simulink model "SoRo_Crt_SMM_20240410"  (R2023a)
settings: Solver=FixedStepAuto  StartTime=0.0  StopTime=50  FixedStep=0.01  RelTol=1e-3
PreLoadFcn:
  | load('traj_pos.mat')
undefined symbols (not defined in the file or in its folder): canChannel
libraries: simulink x18, canmsglib x14, canlib x11, dspfdesign x10, slpidlib x8, auroraNDILibrary x1
(part 2 of 2)

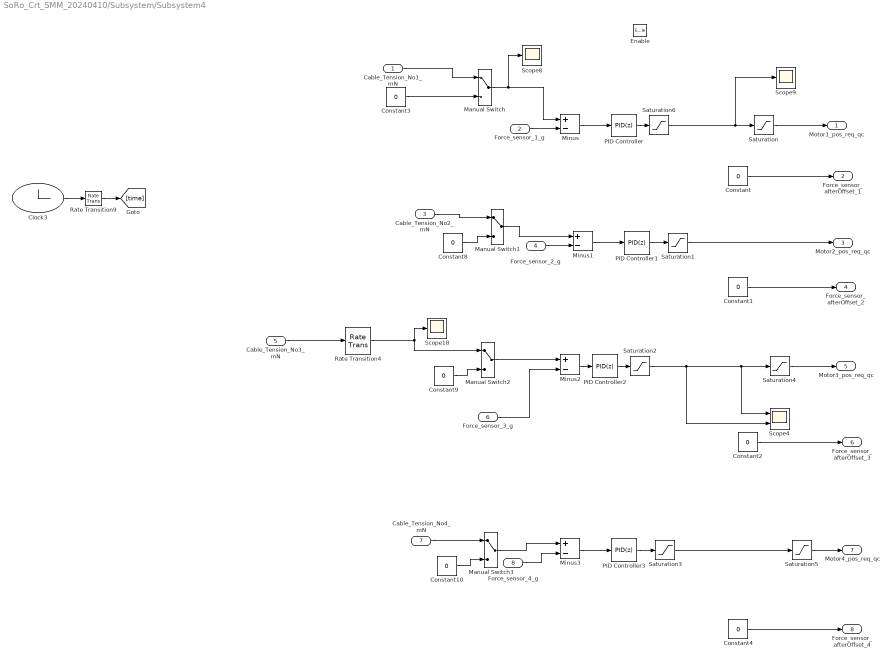
== system SoRo_Crt_SMM_20240410/Subsystem/Subsystem4 ==
  Cable_Tension_No1_mN : Inport
  Force_sensor_1_g : Inport  Port=2
  Cable_Tension_No2_mN : Inport  Port=3
  Force_sensor_2_g : Inport  Port=4
  Cable_Tension_No3_mN : Inport  Port=5
  Force_sensor_3_g : Inport  Port=6
  Cable_Tension_No4_mN : Inport  Port=7
  Force_sensor_4_g : Inport  Port=8
  Enable : EnablePort
  Clock3 : Clock
  Constant{,1..2,4} (4 alike) : Constant  Value=0
  Constant{3,8..10} (4 alike) : Constant  Value=0  SampleTime=0.01
  Manual Switch{,1..3} (4 alike) : ManualSwitch
  Minus{,1..3} (4 alike) : Sum  Inputs=+-
  PID Controller{,1..3} (4 alike) : slpidlib/PID Controller  Controller=PID  Form=Parallel  TimeDomain=Discrete-time  UseExternalTs=off  SampleTime=-1  IntegratorMethod=Forward Euler  FilterMethod=Forward Euler  ControllerParametersSource=internal  P=0.05  I=0.5  UseKiTs=off  D=0  N=100  UseFilter=on  TunerSelectOption=Transfer Function Based (PID Tuner App)  InitialConditionSource=internal  InitialConditionForIntegrator=0  InitialConditionForFilter=0  DifferentiatorICPrevScaledInput=0  ExternalReset=none  TrackingMode=off  Kt=1  LimitOutput=off  SatLimitsSource=internal  UpperSaturationLimit=inf  LowerSaturationLimit=-inf  LinearizeAsGain=on  AntiWindupMode=none  Kb=1  LimitIntegrator=off  UpperIntegratorSaturationLimit=inf  LowerIntegratorSaturationLimit=-inf  POutMin=[]  POutMax=[]  IOutMin=[]  IOutMax=[]  DOutMin=[]  DOutMax=[]  NOutMin=[]  NOutMax=[]  SumOutMin=[]  SumOutMax=[]  SaturationOutMin=[]  SaturationOutMax=[]  PParamMin=[]  PParamMax=[]  IParamMin=[]  IParamMax=[]  DParamMin=[]  DParamMax=[]  NParamMin=[]  NParamMax=[]  KbParamMin=[]  KbParamMax=[]  KtParamMin=[]  KtParamMax=[]  KbOutMin=[]  KbOutMax=[]  KtOutMin=[]  KtOutMax=[]  IntegratorOutMin=[]  IntegratorOutMax=[]  FilterOutMin=[]  FilterOutMax=[]  SumI1OutMin=[]  SumI1OutMax=[]  SumI2OutMin=[]  SumI2OutMax=[]  SumI3OutMin=[]  SumI3OutMax=[]  SumI4OutMin=[]  SumI4OutMax=[]  SumDOutMin=[]  SumDOutMax=[]  DifferentiatorOutMin=[]  DifferentiatorOutMax=[]  FilterDiffOutCoefMin=[]  FilterDiffOutCoefMax=[]  ReciprocalOutMin=[]  ReciprocalOutMax=[]  SumDenOutMin=[]  SumDenOutMax=[]  SumNumOutMin=[]  SumNumOutMax=[]  DivideOutMin=[]  DivideOutMax=[]  UdiffTsProdOutMin=[]  UdiffTsProdOutMax=[]  NTsProdOutMin=[]  NTsProdOutMax=[]  UintegralTsProdOutMin=[]  UintegralTsProdOutMax=[]  UngainTsProdOutMin=[]  UngainTsProdOutMax=[]  ClampingZeroOutDataTypeStr=Inherit: Inherit via back propagation  ClampingZeroOutMin=[]  ClampingZeroOutMax=[]  FilterDenConstantOutDataTypeStr=Inherit: Inherit via back propagation  FilterDenConstantOutMin=[]  FilterDenConstantOutMax=[]  PCopyOutDataTypeStr=Inherit: Inherit via back propagation  PCopyOutMin=[]  PCopyOutMax=[]  NCopyOutDataTypeStr=Inherit: Inherit via back propagation  NCopyOutMin=[]  NCopyOutMax=[]  IntegratorContinuousStateAttributes=''  IntegratorStateMustResolveToSignalObject=off  IntegratorRTWStateStorageClass=Auto  FilterContinuousStateAttributes=''  FilterStateMustResolveToSignalObject=off  FilterRTWStateStorageClass=Auto  ParallelPVariant=InternalParameters  IdealPVariant=Disabled  IVariant=InternalParameters  DVariant=InternalParameters  IntegratorVariant=Discrete  SatVariant=Disabled  AWVariant=Passthrough  PCopyVariant=Disabled  TRVariant=Disabled  FdbkBlocksVariant=Forward  IdealPFdbkVariant=Disabled  SatFdbkVariant=Disabled  DerivativeFilterVariant=ForwardEulerFilter  NVariant=InternalParameters  NCopyVariant=Disabled  FilterICVariant=InternalICsFilter  IntegratorICVariant=InternalICs  ExternalResetVariant=Disabled  TRSumVariant=Passthrough  SumFdbkVariant=Disabled  SumVariant=Sum_PID  TsampFilterVariant=InternalTs  TsampNgainVariant=Passthrough  TsampIntegralVariant=Disabled_SignalSpec  ExternalSaturationOutDataTypeStr=Inherit: Same as second input
  Rate Transition4 : RateTransition  OutPortSampleTime=0.01
  Rate Transition9 : RateTransition  OutPortSampleTime=0.01
  Saturation{,1,4..5} (4 alike) : Saturate  UpperLimit=3000  LowerLimit=-3000
  Saturation2 : Saturate  UpperLimit=400  LowerLimit=-400
  Saturation3 : Saturate  UpperLimit=400  LowerLimit=-400
  Saturation6 : Saturate  UpperLimit=400  LowerLimit=-400
  Scope18 : Scope
  Scope4 : Scope  NumInputPorts=2
  Scope8 : Scope
  Scope9 : Scope
  Motor1_pos_req_qc : Outport
  Force_sensor_afterOffset_1 : Outport  Port=2
  Motor2_pos_req_qc : Outport  Port=3
  Force_sensor_afterOffset_2 : Outport  Port=4
  Motor3_pos_req_qc : Outport  Port=5
  Force_sensor_afterOffset_3 : Outport  Port=6
  Motor4_pos_req_qc : Outport  Port=7
  Force_sensor_afterOffset_4 : Outport  Port=8
  wires:
  Constant8/1 -> Manual Switch1/2
  Minus1/1 -> PID Controller1/1
  PID Controller1/1 -> Saturation1/1
  Manual Switch3/1 -> Minus3/1
  Saturation5/1 -> Motor4_pos_req_qc/1
  PID Controller2/1 -> Saturation2/1
  Saturation4/1 -> Motor3_pos_req_qc/1
  Manual Switch1/1 -> Minus1/1
  Cable_Tension_No4_mN/1 -> Manual Switch3/1
  Manual Switch/1 -> Scope8/1, Minus/1
  Minus3/1 -> PID Controller3/1
  Saturation3/1 -> Saturation5/1
  Manual Switch2/1 -> Minus2/1
  Constant3/1 -> Manual Switch/2
  Cable_Tension_No3_mN/1 -> Rate Transition4/1
  Saturation1/1 -> Motor2_pos_req_qc/1
  Minus/1 -> PID Controller/1
  Constant10/1 -> Manual Switch3/2
  Cable_Tension_No2_mN/1 -> Manual Switch1/1
  Saturation2/1 -> Saturation4/1, Scope4/1, Scope4/2
  PID Controller3/1 -> Saturation3/1
  Saturation/1 -> Motor1_pos_req_qc/1
  PID Controller/1 -> Saturation6/1
  Constant9/1 -> Manual Switch2/2
  Saturation6/1 -> Scope9/1, Saturation/1
  Rate Transition4/1 -> Manual Switch2/1, Scope18/1
  Force_sensor_1_g/1 -> Minus/2
  Force_sensor_3_g/1 -> Minus2/2
  Minus2/1 -> PID Controller2/1
  Force_sensor_2_g/1 -> Minus1/2
  Force_sensor_4_g/1 -> Minus3/2
  Cable_Tension_No1_mN/1 -> Manual Switch/1
  Constant/1 -> Force_sensor_afterOffset_1/1
  Constant1/1 -> Force_sensor_afterOffset_2/1
  Constant2/1 -> Force_sensor_afterOffset_3/1
  Constant4/1 -> Force_sensor_afterOffset_4/1
  Clock3/1 -> Rate Transition9/1
  Rate Transition9/1 -> [time]

== system SoRo_Crt_SMM_20240410/Transmit/Driver_Upload ==
  Enable : EnablePort  StatesWhenEnabling=reset
  CAN Pack_132 : canmsglib/CAN Pack  CANdbFile=E:\Research\SRIL\9th\Mnp_Control_Sim\RoboModule0611.dbc  MsgList=Configuration_all  MsgName=Configuration_all  MsgIDType=Standard (11-bit identifier)  MsgIdentifier=10  MsgLength=8  Remote=off  ApplyMinMax=off  BusOutput=off  SignalInfo={'Data2','16','8','BE','unsigned','Standard','0','1','0','-Inf','Inf';'Data3','24','8','BE','unsigned','Standard','0','1','0','-Inf','Inf';'Data4','32','8','BE','unsigned','Standard','0','1','0','-Inf','Inf';'Data5','40','8','BE','unsigned','Standard','0','1','0','-Inf','Inf';'Data6','48','8','BE','unsigned','Standard','0','1','0','-Inf','Inf';'Data7','56','8','BE','unsigned','Standard','0','1','0','-Inf','Inf';'output_cycle_curvelpos','0','8','BE','unsigned','Standard','0','1','0','-Inf','Inf';'output_cycle_others','8','8','BE','unsigned','Standard','0','1','0','-Inf','Inf'}
      settings: DataFormat=CANdb specified signals
  CAN Transmit : canlib/CAN Transmit  BlockHandle=28690.0002  Device=PEAK-System PCAN-USB (PCAN_USBBUS1)  DeviceMenu=PEAK-System PCAN-USB (PCAN_USBBUS1)  ObjConstructor=canChannel('PEAK-System', 'PCAN_USBBUS1')  EnableEventTransmit=off  EnablePeriodicTransmit=off  MessagePeriod=1.000
  Constant1 : Constant  Value=hex2dec('0x55')  OutDataTypeStr=uint8  SampleTime=-1
  Constant2 : Constant  Value=hex2dec('0x64')  OutDataTypeStr=uint8  SampleTime=-1
  Constant3 : Constant  Value=hex2dec('0x00')  OutDataTypeStr=uint8  SampleTime=-1
  wires:
  Constant1/1 -> CAN Pack_132/3, CAN Pack_132/5, CAN Pack_132/6, CAN Pack_132/4, CAN Pack_132/2, CAN Pack_132/1
  CAN Pack_132/1 -> CAN Transmit/1
  Constant2/1 -> CAN Pack_132/7
  Constant3/1 -> CAN Pack_132/8

== system SoRo_Crt_SMM_20240410/Transmit/Mode Selection ==
  Enable : EnablePort  StatesWhenEnabling=reset
  CAN Pack_132 : canmsglib/CAN Pack  CANdbFile=E:\Research\SRIL\7th\28379Project\Laser_Manipulator_Control\RoboModule.dbc  MsgList=(none)  MsgName=Mode_Selection  MsgIDType=Standard (11-bit identifier)  MsgIdentifier=1  MsgLength=8  Remote=off  ApplyMinMax=off  BusOutput=off  SignalInfo={'Data1','8','8','BE','unsigned','Standard','0','1','0','-Inf','Inf';'Data2','16','8','BE','unsigned','Standard','0','1','0','-Inf','Inf';'Data3','24','8','BE','unsigned','Standard','0','1','0','-Inf','Inf';'Data4','32','8','BE','unsigned','Standard','0','1','0','-Inf','Inf';'Data5','40','8','BE','unsigned','Standard','0','1','0','-Inf','Inf';'Data6','48','8','BE','unsigned','Standard','0','1','0','-Inf','Inf';'Data7','56','8','BE','unsigned','Standard','0','1','0','-Inf','Inf';'Mode','0','8','BE','unsigned','Standard','0','1','0','-Inf','Inf'}
      settings: DataFormat=CANdb specified signals
  CAN Transmit : canlib/CAN Transmit  BlockHandle=28790.0002  Device=PEAK-System PCAN-USB (PCAN_USBBUS1)  DeviceMenu=PEAK-System PCAN-USB (PCAN_USBBUS1)  ObjConstructor=canChannel('PEAK-System', 'PCAN_USBBUS1')  EnableEventTransmit=off  EnablePeriodicTransmit=off  MessagePeriod=1.000
  Constant1 : Constant  Value=hex2dec('0x55')  OutDataTypeStr=uint8  SampleTime=-1
  Mode Number : Constant  Value=hex2dec('0x04')  OutDataTypeStr=uint8  SampleTime=-1
  wires:
  CAN Pack_132/1 -> CAN Transmit/1
  Constant1/1 -> CAN Pack_132/7, CAN Pack_132/6, CAN Pack_132/5, CAN Pack_132/4, CAN Pack_132/3, CAN Pack_132/2, CAN Pack_132/1
  Mode Number/1 -> CAN Pack_132/8

== system SoRo_Crt_SMM_20240410/Transmit/PosSpdMode1 ==
  note: R ated Voltage of Motor is 12 V. Supply Voltage is 24 V. Limilation of the temp_pwm is set as 2500.
  Inport1 : Inport
  Enable : EnablePort
  Add : Sum
  CAN Pack_132 : canmsglib/CAN Pack  CANdbFile=E:\Research\SRIL\9th\Mnp_Control_Sim\RoboModule0611.dbc  MsgList=Position_Dr1  MsgName=Position_Dr1  MsgIDType=Standard (11-bit identifier)  MsgIdentifier=21  MsgLength=8  Remote=off  ApplyMinMax=off  BusOutput=off  SignalInfo={'Data2','16','8','BE','unsigned','Standard','0','1','0','-Inf','Inf';'Data3','24','8','BE','unsigned','Standard','0','1','0','-Inf','Inf';'temp_position','56','32','BE','signed','Standard','0','1','0','-Inf','Inf';'temp_pwm','8','16','BE','unsigned','Standard','0','1','0','-Inf','Inf'}
      settings: DataFormat=CANdb specified signals
  CAN Transmit : canlib/CAN Transmit  BlockHandle=28846.0002  Device=PEAK-System PCAN-USB (PCAN_USBBUS1)  DeviceMenu=PEAK-System PCAN-USB (PCAN_USBBUS1)  ObjConstructor=canChannel('PEAK-System', 'PCAN_USBBUS1')  EnableEventTransmit=off  EnablePeriodicTransmit=on  MessagePeriod=0.01
  Constant : Constant  Value=5000
  Constant1 : Constant
  Constant2 : Constant  Value=hex2dec('0x55')  OutDataTypeStr=uint8  SampleTime=-1
  Delay : Delay  DelayLength=1
  flag : Outport
  wires:
  CAN Pack_132/1 -> CAN Transmit/1
  Inport1/1 -> CAN Pack_132/3
  Constant1/1 -> Add/1
  Add/1 -> Delay/1, flag/1
  Delay/1 -> Add/2
  Constant2/1 -> CAN Pack_132/2, CAN Pack_132/1
  Constant/1 -> CAN Pack_132/4

== system SoRo_Crt_SMM_20240410/Transmit/PosSpdMode2 ==
  note: R ated Voltage of Motor is 12 V. Supply Voltage is 24 V. Limilation of the temp_pwm is set as 2500.
  Inport1 : Inport
  Enable : EnablePort
  Add : Sum
  CAN Pack_132 : canmsglib/CAN Pack  CANdbFile=E:\Research\SRIL\9th\Mnp_Control_Sim\RoboModule0611.dbc  MsgList=Position_Dr2  MsgName=Position_Dr2  MsgIDType=Standard (11-bit identifier)  MsgIdentifier=37  MsgLength=8  Remote=off  ApplyMinMax=off  BusOutput=off  SignalInfo={'Data2','16','8','BE','unsigned','Standard','0','1','0','-Inf','Inf';'Data3','24','8','BE','unsigned','Standard','0','1','0','-Inf','Inf';'temp_position','56','32','BE','signed','Standard','0','1','0','-Inf','Inf';'temp_pwm','8','16','BE','unsigned','Standard','0','1','0','-Inf','Inf'}
      settings: DataFormat=CANdb specified signals
  CAN Transmit : canlib/CAN Transmit  BlockHandle=28896.0002  Device=PEAK-System PCAN-USB (PCAN_USBBUS1)  DeviceMenu=PEAK-System PCAN-USB (PCAN_USBBUS1)  ObjConstructor=canChannel('PEAK-System', 'PCAN_USBBUS1')  EnableEventTransmit=off  EnablePeriodicTransmit=on  MessagePeriod=0.01
  Constant : Constant  Value=5000
  Constant1 : Constant
  Constant2 : Constant  Value=hex2dec('0x55')  OutDataTypeStr=uint8  SampleTime=-1
  Delay : Delay  DelayLength=1
  flag : Outport
  wires:
  CAN Pack_132/1 -> CAN Transmit/1
  Inport1/1 -> CAN Pack_132/3
  Constant1/1 -> Add/1
  Add/1 -> Delay/1, flag/1
  Delay/1 -> Add/2
  Constant2/1 -> CAN Pack_132/2, CAN Pack_132/1
  Constant/1 -> CAN Pack_132/4

== system SoRo_Crt_SMM_20240410/Transmit/PosSpdMode3 ==
  note: R ated Voltage of Motor is 12 V. Supply Voltage is 24 V. Limilation of the temp_pwm is set as 2500.
  Inport1 : Inport
  Enable : EnablePort
  Add : Sum
  CAN Pack_132 : canmsglib/CAN Pack  CANdbFile=E:\Research\SRIL\9th\Mnp_Control_Sim\RoboModule0611.dbc  MsgList=Position_Dr3  MsgName=Position_Dr3  MsgIDType=Standard (11-bit identifier)  MsgIdentifier=53  MsgLength=8  Remote=off  ApplyMinMax=off  BusOutput=off  SignalInfo={'Data2','16','8','BE','unsigned','Standard','0','1','0','-Inf','Inf';'Data3','24','8','BE','unsigned','Standard','0','1','0','-Inf','Inf';'temp_position','56','32','BE','signed','Standard','0','1','0','-Inf','Inf';'temp_pwm','8','16','BE','unsigned','Standard','0','1','0','-Inf','Inf'}
      settings: DataFormat=CANdb specified signals
  CAN Transmit : canlib/CAN Transmit  BlockHandle=28962.0002  Device=PEAK-System PCAN-USB (PCAN_USBBUS1)  DeviceMenu=PEAK-System PCAN-USB (PCAN_USBBUS1)  ObjConstructor=canChannel('PEAK-System', 'PCAN_USBBUS1')  EnableEventTransmit=off  EnablePeriodicTransmit=on  MessagePeriod=0.01
  Constant : Constant  Value=5000
  Constant1 : Constant
  Constant2 : Constant  Value=hex2dec('0x55')  OutDataTypeStr=uint8  SampleTime=-1
  Delay : Delay  DelayLength=1
  flag : Outport
  wires:
  CAN Pack_132/1 -> CAN Transmit/1
  Inport1/1 -> CAN Pack_132/3
  Constant1/1 -> Add/1
  Add/1 -> Delay/1, flag/1
  Delay/1 -> Add/2
  Constant2/1 -> CAN Pack_132/2, CAN Pack_132/1
  Constant/1 -> CAN Pack_132/4

== system SoRo_Crt_SMM_20240410/Transmit/PosSpdMode4 ==
  note: R ated Voltage of Motor is 12 V. Supply Voltage is 24 V. Limilation of the temp_pwm is set as 2500.
  Inport1 : Inport
  Enable : EnablePort
  Add : Sum
  CAN Pack_132 : canmsglib/CAN Pack  CANdbFile=E:\Research\SRIL\9th\Mnp_Control_Sim\RoboModule0611.dbc  MsgList=Position_Dr4  MsgName=Position_Dr4  MsgIDType=Standard (11-bit identifier)  MsgIdentifier=69  MsgLength=8  Remote=off  ApplyMinMax=off  BusOutput=off  SignalInfo={'Data2','16','8','BE','unsigned','Standard','0','1','0','-Inf','Inf';'Data3','24','8','BE','unsigned','Standard','0','1','0','-Inf','Inf';'temp_position','56','32','BE','signed','Standard','0','1','0','-Inf','Inf';'temp_pwm','8','16','BE','unsigned','Standard','0','1','0','-Inf','Inf'}
      settings: DataFormat=CANdb specified signals
  CAN Transmit : canlib/CAN Transmit  BlockHandle=29015.0002  Device=PEAK-System PCAN-USB (PCAN_USBBUS1)  DeviceMenu=PEAK-System PCAN-USB (PCAN_USBBUS1)  ObjConstructor=canChannel('PEAK-System', 'PCAN_USBBUS1')  EnableEventTransmit=off  EnablePeriodicTransmit=on  MessagePeriod=0.01
  Constant : Constant  Value=5000
  Constant1 : Constant
  Constant2 : Constant  Value=hex2dec('0x55')  OutDataTypeStr=uint8  SampleTime=-1
  Delay : Delay  DelayLength=1
  flag : Outport
  wires:
  CAN Pack_132/1 -> CAN Transmit/1
  Inport1/1 -> CAN Pack_132/3
  Constant1/1 -> Add/1
  Add/1 -> Delay/1, flag/1
  Delay/1 -> Add/2
  Constant2/1 -> CAN Pack_132/2, CAN Pack_132/1
  Constant/1 -> CAN Pack_132/4

== system SoRo_Crt_SMM_20240410/Transmit/Reset ==
  Enable : EnablePort  StatesWhenEnabling=reset
  CAN Pack_132 : canmsglib/CAN Pack  CANdbFile=E:\Research\SRIL\7th\28379Project\Laser_Manipulator_Control\RoboModule.dbc  MsgList=(none)  MsgName=Reset  MsgIDType=Standard (11-bit identifier)  MsgIdentifier=0  MsgLength=8  Remote=off  ApplyMinMax=off  BusOutput=off  SignalInfo={'Data0','0','8','BE','unsigned','Standard','0','1','0','-Inf','Inf';'Data1','8','8','BE','unsigned','Standard','0','1','0','-Inf','Inf';'Data2','16','8','BE','unsigned','Standard','0','1','0','-Inf','Inf';'Data3','24','8','BE','unsigned','Standard','0','1','0','-Inf','Inf';'Data4','32','8','BE','unsigned','Standard','0','1','0','-Inf','Inf';'Data5','40','8','BE','unsigned','Standard','0','1','0','-Inf','Inf';'Data6','48','8','BE','unsigned','Standard','0','1','0','-Inf','Inf';'Data7','56','8','BE','unsigned','Standard','0','1','0','-Inf','Inf'}
      settings: DataFormat=CANdb specified signals
  CAN Transmit : canlib/CAN Transmit  BlockHandle=29087.0002  Device=PEAK-System PCAN-USB (PCAN_USBBUS1)  DeviceMenu=PEAK-System PCAN-USB (PCAN_USBBUS1)  ObjConstructor=canChannel('PEAK-System', 'PCAN_USBBUS1')  EnableEventTransmit=off  EnablePeriodicTransmit=off  MessagePeriod=1.000
  Constant1 : Constant  Value=hex2dec('0x55')  OutDataTypeStr=uint8  SampleTime=-1
  wires:
  Constant1/1 -> CAN Pack_132/3, CAN Pack_132/5, CAN Pack_132/6, CAN Pack_132/7, CAN Pack_132/8, CAN Pack_132/4, CAN Pack_132/2, CAN Pack_132/1
  CAN Pack_132/1 -> CAN Transmit/1

== system SoRo_Crt_SMM_20240410/Transmit/Reset1 ==
  Enable : EnablePort  StatesWhenEnabling=reset
  CAN Pack_132 : canmsglib/CAN Pack  CANdbFile=E:\Research\SRIL\7th\28379Project\Laser_Manipulator_Control\RoboModule.dbc  MsgList=(none)  MsgName=Reset  MsgIDType=Standard (11-bit identifier)  MsgIdentifier=0  MsgLength=8  Remote=off  ApplyMinMax=off  BusOutput=off  SignalInfo={'Data0','0','8','BE','unsigned','Standard','0','1','0','-Inf','Inf';'Data1','8','8','BE','unsigned','Standard','0','1','0','-Inf','Inf';'Data2','16','8','BE','unsigned','Standard','0','1','0','-Inf','Inf';'Data3','24','8','BE','unsigned','Standard','0','1','0','-Inf','Inf';'Data4','32','8','BE','unsigned','Standard','0','1','0','-Inf','Inf';'Data5','40','8','BE','unsigned','Standard','0','1','0','-Inf','Inf';'Data6','48','8','BE','unsigned','Standard','0','1','0','-Inf','Inf';'Data7','56','8','BE','unsigned','Standard','0','1','0','-Inf','Inf'}
      settings: DataFormat=CANdb specified signals
  CAN Transmit : canlib/CAN Transmit  BlockHandle=29145.0002  Device=PEAK-System PCAN-USB (PCAN_USBBUS1)  DeviceMenu=PEAK-System PCAN-USB (PCAN_USBBUS1)  ObjConstructor=canChannel('PEAK-System', 'PCAN_USBBUS1')  EnableEventTransmit=off  EnablePeriodicTransmit=off  MessagePeriod=1.000
  Constant1 : Constant  Value=hex2dec('0x55')  OutDataTypeStr=uint8  SampleTime=-1
  wires:
  Constant1/1 -> CAN Pack_132/3, CAN Pack_132/5, CAN Pack_132/6, CAN Pack_132/7, CAN Pack_132/8, CAN Pack_132/4, CAN Pack_132/2, CAN Pack_132/1
  CAN Pack_132/1 -> CAN Transmit/1

== system SoRo_Crt_SMM_20240410/Transmit/Reset_Manually ==
  Enable : EnablePort  StatesWhenEnabling=reset
  Trigger : TriggerPort  VariantControl=(inherit)  PortDimensions=1
  CAN Pack_132 : canmsglib/CAN Pack  CANdbFile=E:\Research\SRIL\9th\Mnp_Control_Sim\RoboModule0611.dbc  MsgList=Reset_all  MsgName=Reset_all  MsgIDType=Standard (11-bit identifier)  MsgIdentifier=0  MsgLength=8  Remote=off  ApplyMinMax=off  BusOutput=off  SignalInfo={'Data0','0','8','BE','unsigned','Standard','0','1','0','-Inf','Inf';'Data1','8','8','BE','unsigned','Standard','0','1','0','-Inf','Inf';'Data2','16','8','BE','unsigned','Standard','0','1','0','-Inf','Inf';'Data3','24','8','BE','unsigned','Standard','0','1','0','-Inf','Inf';'Data4','32','8','BE','unsigned','Standard','0','1','0','-Inf','Inf';'Data5','40','8','BE','unsigned','Standard','0','1','0','-Inf','Inf';'Data6','48','8','BE','unsigned','Standard','0','1','0','-Inf','Inf';'Data7','56','8','BE','unsigned','Standard','0','1','0','-Inf','Inf'}
      settings: DataFormat=CANdb specified signals
  CAN Transmit : canlib/CAN Transmit  BlockHandle=29200.0002  Device=PEAK-System PCAN-USB (PCAN_USBBUS1)  DeviceMenu=PEAK-System PCAN-USB (PCAN_USBBUS1)  ObjConstructor=canChannel('PEAK-System', 'PCAN_USBBUS1')  EnableEventTransmit=off  EnablePeriodicTransmit=off  MessagePeriod=1.000
  Constant1 : Constant  Value=hex2dec('0x55')  OutDataTypeStr=uint8  SampleTime=-1
  wires:
  CAN Pack_132/1 -> CAN Transmit/1
  Constant1/1 -> CAN Pack_132/1, CAN Pack_132/2, CAN Pack_132/4, CAN Pack_132/8, CAN Pack_132/7, CAN Pack_132/6, CAN Pack_132/5, CAN Pack_132/3

== system SoRo_Crt_SMM_20240410/Aurora/Subsystem4/Subsystem ==
  In1 : Inport
  Enable : EnablePort
  Analog Filter Design{1..5,11} (6 alike) : dspfdesign/Analog Filter Design  method=Chebyshev I  filttype=Lowpass  N=3  Wlo=10  Whi=80  Rp=2  Rs=40
  Demux : Demux  Outputs=6
  Mux1 : Mux  Inputs=6
  Scope3 : Scope  NumInputPorts=2
  Out1 : Outport
  wires:
  Analog Filter Design1/1 -> Mux1/2
  Demux/1 -> Analog Filter Design11/1
  Analog Filter Design2/1 -> Mux1/3
  Demux/3 -> Analog Filter Design2/1
  Demux/6 -> Scope3/2, Analog Filter Design5/1
  Analog Filter Design3/1 -> Mux1/4
  Demux/5 -> Analog Filter Design4/1
  Analog Filter Design5/1 -> Scope3/1, Mux1/6
  Demux/4 -> Analog Filter Design3/1
  Mux1/1 -> Out1/1
  Analog Filter Design11/1 -> Mux1/1
  Analog Filter Design4/1 -> Mux1/5
  Demux/2 -> Analog Filter Design1/1
  In1/1 -> Demux/1

== system SoRo_Crt_SMM_20240410/Aurora/Subsystem4/Subsystem1 ==
  encoder1 : Inport
  Enable : EnablePort
  Add : Sum  Inputs=+-
  Constant : Constant  Value=[0.1522,0.0345,-0.1449,0.1476,0.0344,-0.1416]
  Scope1 : Scope
  Scope2 : Scope
  Out1 : Outport
  wires:
  encoder1/1 -> Scope2/1, Add/1
  Add/1 -> Out1/1
  Constant/1 -> Scope1/1, Add/2

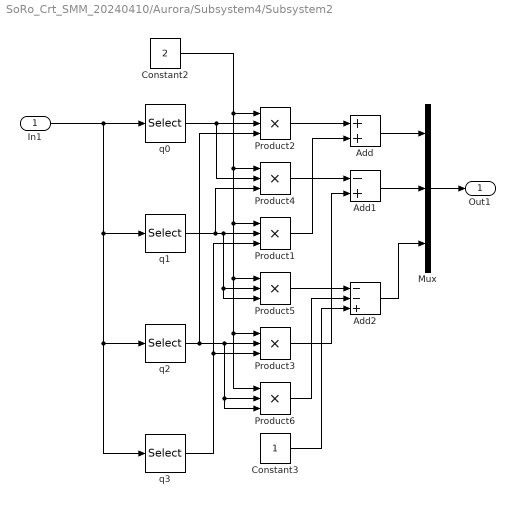
== system SoRo_Crt_SMM_20240410/Aurora/Subsystem4/Subsystem2 ==
  In1 : Inport
  Add : Sum
  Add1 : Sum  Inputs=-+
  Add2 : Sum  Inputs=--+
  Constant2 : Constant  Value=2
  Constant3 : Constant
  Mux : Mux  Inputs=3
  Product{1..6} (6 alike) : Product  Inputs=3
  q0 : Selector  InputPortWidth=4  IndexOptions=Index vector (dialog)  Indices=[1]  OutputSizes=1
  q1 : Selector  InputPortWidth=4  IndexOptions=Index vector (dialog)  Indices=[2]  OutputSizes=1
  q2 : Selector  InputPortWidth=4  IndexOptions=Index vector (dialog)  Indices=[3]  OutputSizes=1
  q3 : Selector  InputPortWidth=4  IndexOptions=Index vector (dialog)  Indices=[4]  OutputSizes=1
  Out1 : Outport
  wires:
  Product2/1 -> Add/1
  Constant2/1 -> Product4/1, Product5/1, Product3/1, Product6/1, Product1/1, Product2/1
  Add/1 -> Mux/1
  q2/1 -> Product6/3, Product6/2, Product3/2, Product2/3
  q1/1 -> Product4/3, Product5/3, Product5/2, Product1/2
  q3/1 -> Product3/3, Product1/3
  q0/1 -> Product4/2, Product2/2
  Product3/1 -> Add1/2
  Add1/1 -> Mux/2
  In1/1 -> q1/1, q2/1, q3/1, q0/1
  Add2/1 -> Mux/3
  Constant3/1 -> Add2/3
  Product1/1 -> Add/2
  Product5/1 -> Add2/1
  Product6/1 -> Add2/2
  Product4/1 -> Add1/1
  Mux/1 -> Out1/1

== system SoRo_Crt_SMM_20240410/Aurora/Subsystem5/Subsystem2 ==
  In1 : Inport
  Matrix Concatenate : Concatenate  NumInputs=3  Mode=Multidimensional array  ConcatenateDimension=2
  Subsystem1 : Subsystem
      mask Display: disp('y vector');
  Subsystem2 : Subsystem
      mask Display: disp('z vector');
  Subsystem3 : Subsystem
      mask Display: disp('x vector');
  Out1 : Outport
  wires:
  In1/1 -> Subsystem1/1(In1), Subsystem2/1(In1), Subsystem3/1(In1)
  Matrix Concatenate/1 -> Out1/1
  Subsystem3/1(Out1) -> Matrix Concatenate/1
  Subsystem1/1(Out1) -> Matrix Concatenate/2
  Subsystem2/1(Out1) -> Matrix Concatenate/3

== system SoRo_Crt_SMM_20240410/Aurora/Subsystem5/Subsystem3 ==
  In1 : Inport
  Matrix Concatenate : Concatenate  NumInputs=3  Mode=Multidimensional array  ConcatenateDimension=2
  Subsystem1 : Subsystem
      mask Display: disp('y vector');
  Subsystem2 : Subsystem
      mask Display: disp('z vector');
  Subsystem3 : Subsystem
      mask Display: disp('x vector');
  Out1 : Outport
  wires:
  Subsystem2/1(Out1) -> Matrix Concatenate/3
  Subsystem1/1(Out1) -> Matrix Concatenate/2
  Subsystem3/1(Out1) -> Matrix Concatenate/1
  Matrix Concatenate/1 -> Out1/1
  In1/1 -> Subsystem3/1(In1), Subsystem2/1(In1), Subsystem1/1(In1)

== system SoRo_Crt_SMM_20240410/Subsystem/Subsystem1/Subsystem ==
  encoder1 : Inport
  Enable : EnablePort
  Out1 : Outport
  wires:
  encoder1/1 -> Out1/1

== system SoRo_Crt_SMM_20240410/Subsystem/Subsystem1/Subsystem1 ==
  encoder1 : Inport
  Enable : EnablePort
  Out1 : Outport
  wires:
  encoder1/1 -> Out1/1

== system SoRo_Crt_SMM_20240410/Subsystem/Subsystem1/Subsystem2 ==
  encoder1 : Inport
  Enable : EnablePort
  Out1 : Outport
  wires:
  encoder1/1 -> Out1/1

== system SoRo_Crt_SMM_20240410/Subsystem/Subsystem1/Subsystem3 ==
  encoder1 : Inport
  Enable : EnablePort
  Out1 : Outport
  wires:
  encoder1/1 -> Out1/1

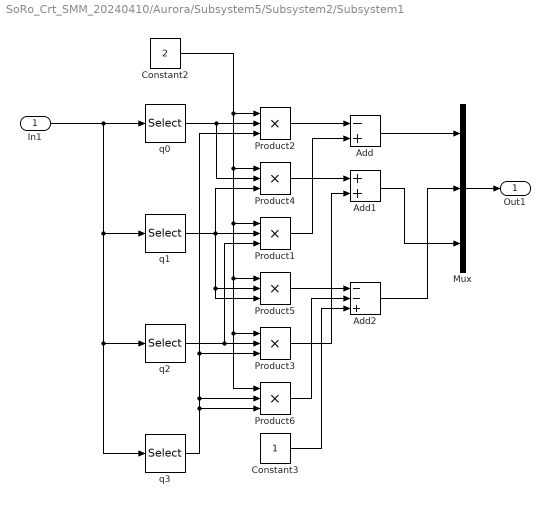
== system SoRo_Crt_SMM_20240410/Aurora/Subsystem5/Subsystem2/Subsystem1 ==
  In1 : Inport
  Add : Sum  Inputs=-+
  Add1 : Sum
  Add2 : Sum  Inputs=--+
  Constant2 : Constant  Value=2
  Constant3 : Constant
  Mux : Mux  Inputs=3
  Product{1..6} (6 alike) : Product  Inputs=3
  q0 : Selector  InputPortWidth=4  IndexOptions=Index vector (dialog)  Indices=[1]  OutputSizes=1
  q1 : Selector  InputPortWidth=4  IndexOptions=Index vector (dialog)  Indices=[2]  OutputSizes=1
  q2 : Selector  InputPortWidth=4  IndexOptions=Index vector (dialog)  Indices=[3]  OutputSizes=1
  q3 : Selector  InputPortWidth=4  IndexOptions=Index vector (dialog)  Indices=[4]  OutputSizes=1
  Out1 : Outport
  wires:
  Mux/1 -> Out1/1
  Product4/1 -> Add1/1
  Product6/1 -> Add2/2
  Product5/1 -> Add2/1
  Product1/1 -> Add/2
  Constant3/1 -> Add2/3
  Add2/1 -> Mux/2
  In1/1 -> q0/1, q3/1, q2/1, q1/1
  Add1/1 -> Mux/3
  Product3/1 -> Add1/2
  q0/1 -> Product2/2, Product4/2
  q3/1 -> Product3/3, Product2/3, Product6/2, Product6/3
  q1/1 -> Product1/2, Product5/2, Product5/3, Product4/3
  q2/1 -> Product1/3, Product3/2
  Add/1 -> Mux/1
  Constant2/1 -> Product2/1, Product1/1, Product6/1, Product3/1, Product5/1, Product4/1
  Product2/1 -> Add/1

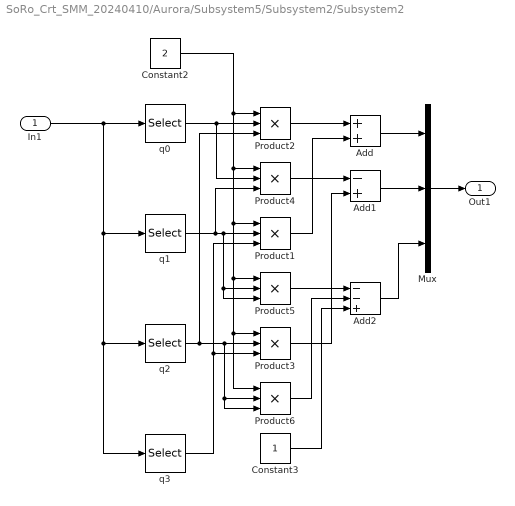
== system SoRo_Crt_SMM_20240410/Aurora/Subsystem5/Subsystem2/Subsystem2 ==
  In1 : Inport
  Add : Sum
  Add1 : Sum  Inputs=-+
  Add2 : Sum  Inputs=--+
  Constant2 : Constant  Value=2
  Constant3 : Constant
  Mux : Mux  Inputs=3
  Product{1..6} (6 alike) : Product  Inputs=3
  q0 : Selector  InputPortWidth=4  IndexOptions=Index vector (dialog)  Indices=[1]  OutputSizes=1
  q1 : Selector  InputPortWidth=4  IndexOptions=Index vector (dialog)  Indices=[2]  OutputSizes=1
  q2 : Selector  InputPortWidth=4  IndexOptions=Index vector (dialog)  Indices=[3]  OutputSizes=1
  q3 : Selector  InputPortWidth=4  IndexOptions=Index vector (dialog)  Indices=[4]  OutputSizes=1
  Out1 : Outport
  wires:
  Product2/1 -> Add/1
  Constant2/1 -> Product4/1, Product5/1, Product3/1, Product6/1, Product1/1, Product2/1
  Add/1 -> Mux/1
  q2/1 -> Product6/3, Product6/2, Product3/2, Product2/3
  q1/1 -> Product4/3, Product5/3, Product5/2, Product1/2
  q3/1 -> Product3/3, Product1/3
  q0/1 -> Product4/2, Product2/2
  Product3/1 -> Add1/2
  Add1/1 -> Mux/2
  In1/1 -> q1/1, q2/1, q3/1, q0/1
  Add2/1 -> Mux/3
  Constant3/1 -> Add2/3
  Product1/1 -> Add/2
  Product5/1 -> Add2/1
  Product6/1 -> Add2/2
  Product4/1 -> Add1/1
  Mux/1 -> Out1/1

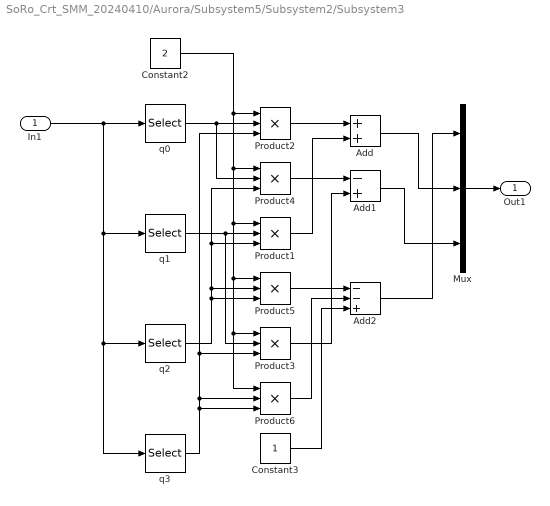
== system SoRo_Crt_SMM_20240410/Aurora/Subsystem5/Subsystem2/Subsystem3 ==
  In1 : Inport
  Add : Sum
  Add1 : Sum  Inputs=-+
  Add2 : Sum  Inputs=--+
  Constant2 : Constant  Value=2
  Constant3 : Constant
  Mux : Mux  Inputs=3
  Product{1..6} (6 alike) : Product  Inputs=3
  q0 : Selector  InputPortWidth=4  IndexOptions=Index vector (dialog)  Indices=[1]  OutputSizes=1
  q1 : Selector  InputPortWidth=4  IndexOptions=Index vector (dialog)  Indices=[2]  OutputSizes=1
  q2 : Selector  InputPortWidth=4  IndexOptions=Index vector (dialog)  Indices=[3]  OutputSizes=1
  q3 : Selector  InputPortWidth=4  IndexOptions=Index vector (dialog)  Indices=[4]  OutputSizes=1
  Out1 : Outport
  wires:
  Product2/1 -> Add/1
  Constant2/1 -> Product4/1, Product5/1, Product3/1, Product6/1, Product1/1, Product2/1
  Add/1 -> Mux/2
  q2/1 -> Product5/3, Product5/2, Product1/3, Product4/3
  q1/1 -> Product3/2, Product1/2
  q3/1 -> Product6/3, Product6/2, Product2/3, Product3/3
  q0/1 -> Product4/2, Product2/2
  Product3/1 -> Add1/2
  Add1/1 -> Mux/3
  In1/1 -> q1/1, q2/1, q3/1, q0/1
  Add2/1 -> Mux/1
  Constant3/1 -> Add2/3
  Product1/1 -> Add/2
  Product5/1 -> Add2/1
  Product6/1 -> Add2/2
  Product4/1 -> Add1/1
  Mux/1 -> Out1/1

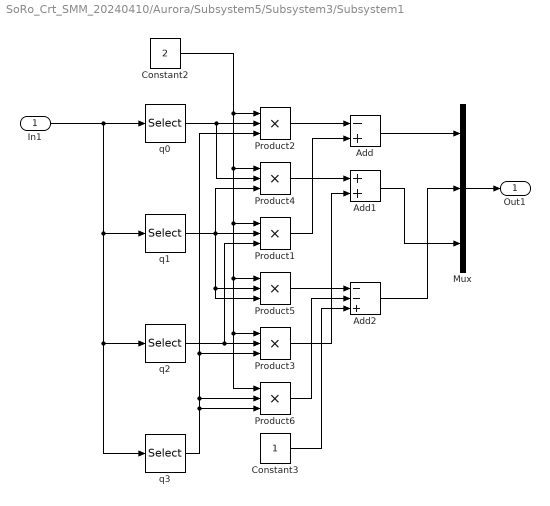
== system SoRo_Crt_SMM_20240410/Aurora/Subsystem5/Subsystem3/Subsystem1 ==
  In1 : Inport
  Add : Sum  Inputs=-+
  Add1 : Sum
  Add2 : Sum  Inputs=--+
  Constant2 : Constant  Value=2
  Constant3 : Constant
  Mux : Mux  Inputs=3
  Product{1..6} (6 alike) : Product  Inputs=3
  q0 : Selector  InputPortWidth=4  IndexOptions=Index vector (dialog)  Indices=[1]  OutputSizes=1
  q1 : Selector  InputPortWidth=4  IndexOptions=Index vector (dialog)  Indices=[2]  OutputSizes=1
  q2 : Selector  InputPortWidth=4  IndexOptions=Index vector (dialog)  Indices=[3]  OutputSizes=1
  q3 : Selector  InputPortWidth=4  IndexOptions=Index vector (dialog)  Indices=[4]  OutputSizes=1
  Out1 : Outport
  wires:
  Product2/1 -> Add/1
  Constant2/1 -> Product4/1, Product5/1, Product3/1, Product6/1, Product1/1, Product2/1
  Add/1 -> Mux/1
  q2/1 -> Product3/2, Product1/3
  q1/1 -> Product4/3, Product5/3, Product5/2, Product1/2
  q3/1 -> Product6/3, Product6/2, Product2/3, Product3/3
  q0/1 -> Product4/2, Product2/2
  Product3/1 -> Add1/2
  Add1/1 -> Mux/3
  In1/1 -> q1/1, q2/1, q3/1, q0/1
  Add2/1 -> Mux/2
  Constant3/1 -> Add2/3
  Product1/1 -> Add/2
  Product5/1 -> Add2/1
  Product6/1 -> Add2/2
  Product4/1 -> Add1/1
  Mux/1 -> Out1/1

== system SoRo_Crt_SMM_20240410/Aurora/Subsystem5/Subsystem3/Subsystem2 ==
  In1 : Inport
  Add : Sum
  Add1 : Sum  Inputs=-+
  Add2 : Sum  Inputs=--+
  Constant2 : Constant  Value=2
  Constant3 : Constant
  Mux : Mux  Inputs=3
  Product{1..6} (6 alike) : Product  Inputs=3
  q0 : Selector  InputPortWidth=4  IndexOptions=Index vector (dialog)  Indices=[1]  OutputSizes=1
  q1 : Selector  InputPortWidth=4  IndexOptions=Index vector (dialog)  Indices=[2]  OutputSizes=1
  q2 : Selector  InputPortWidth=4  IndexOptions=Index vector (dialog)  Indices=[3]  OutputSizes=1
  q3 : Selector  InputPortWidth=4  IndexOptions=Index vector (dialog)  Indices=[4]  OutputSizes=1
  Out1 : Outport
  wires:
  Mux/1 -> Out1/1
  Product4/1 -> Add1/1
  Product6/1 -> Add2/2
  Product5/1 -> Add2/1
  Product1/1 -> Add/2
  Constant3/1 -> Add2/3
  Add2/1 -> Mux/3
  In1/1 -> q0/1, q3/1, q2/1, q1/1
  Add1/1 -> Mux/2
  Product3/1 -> Add1/2
  q0/1 -> Product2/2, Product4/2
  q3/1 -> Product1/3, Product3/3
  q1/1 -> Product1/2, Product5/2, Product5/3, Product4/3
  q2/1 -> Product2/3, Product3/2, Product6/2, Product6/3
  Add/1 -> Mux/1
  Constant2/1 -> Product2/1, Product1/1, Product6/1, Product3/1, Product5/1, Product4/1
  Product2/1 -> Add/1

== system SoRo_Crt_SMM_20240410/Aurora/Subsystem5/Subsystem3/Subsystem3 ==
  In1 : Inport
  Add : Sum
  Add1 : Sum  Inputs=-+
  Add2 : Sum  Inputs=--+
  Constant2 : Constant  Value=2
  Constant3 : Constant
  Mux : Mux  Inputs=3
  Product{1..6} (6 alike) : Product  Inputs=3
  q0 : Selector  InputPortWidth=4  IndexOptions=Index vector (dialog)  Indices=[1]  OutputSizes=1
  q1 : Selector  InputPortWidth=4  IndexOptions=Index vector (dialog)  Indices=[2]  OutputSizes=1
  q2 : Selector  InputPortWidth=4  IndexOptions=Index vector (dialog)  Indices=[3]  OutputSizes=1
  q3 : Selector  InputPortWidth=4  IndexOptions=Index vector (dialog)  Indices=[4]  OutputSizes=1
  Out1 : Outport
  wires:
  Mux/1 -> Out1/1
  Product4/1 -> Add1/1
  Product6/1 -> Add2/2
  Product5/1 -> Add2/1
  Product1/1 -> Add/2
  Constant3/1 -> Add2/3
  Add2/1 -> Mux/1
  In1/1 -> q0/1, q3/1, q2/1, q1/1
  Add1/1 -> Mux/3
  Product3/1 -> Add1/2
  q0/1 -> Product2/2, Product4/2
  q3/1 -> Product3/3, Product2/3, Product6/2, Product6/3
  q1/1 -> Product1/2, Product3/2
  q2/1 -> Product4/3, Product1/3, Product5/2, Product5/3
  Add/1 -> Mux/2
  Constant2/1 -> Product2/1, Product1/1, Product6/1, Product3/1, Product5/1, Product4/1
  Product2/1 -> Add/1

== matlab function SoRo_Crt_SMM_20240410/Aurora/Subsystem4/MATLAB Function1 ==
  data: DataEqm output; Orien5dof_z input; DOF6 input; OrgData output; eqm input; Dof6Last input
function [DataEqm,OrgData] = dataAssemble( Orien5dof_z, DOF6, eqm, Dof6Last )
Dof6Filter = DOF6;
if eqm(1) > 0
    for i = 1:3
        if abs(DOF6(i) - Dof6Last(i)) > 0.5
            Dof6Filter(i) =  Dof6Last(i);
        end
    end
end
SecPot = Dof6Filter + Orien5dof_z;
OrgData = [SecPot;Dof6Filter];
DataEqmFull = OrgData-eqm;
DataEqm = DataEqmFull(4:6);
end

== matlab function SoRo_Crt_SMM_20240410/SQP ==
  settings: updateMethod=DISCRETE  sampleTime=0.05
  data: trq_right_1_last input; trq_btm_2_last input; trq_top_3_last input; trq_left_4_last input; trq_right_1 output; trq_btm_2 output; dataAss input; trq_top_3 output; time input; z_warm input; trq_left_4 output; flag output; x_0 output; trq_right_1_ori output; trq_btm_2_ori output; trq_top_3_ori output; trq_left_4_ori output; pos data_store_memory; vel data_store_memory; z_last output size=[80]
function [trq_right_1,trq_btm_2,trq_top_3,trq_left_4,flag, x_0,trq_right_1_ori,trq_btm_2_ori,trq_top_3_ori,trq_left_4_ori,z_last] = fcn(trq_right_1_last,trq_btm_2_last,trq_top_3_last,trq_left_4_last,dataAss,time,z_warm)
% Returns the calculated control action (required cable tension). They are
% the first control action from the calculated control sequence with MPC
% scheme.
%
% INPUT
% tip_pos_orie - vector of dimension (6,1) where the first element
%                represents the bending angle and the next two elements
%                represent the normolized bending direction projected to
%                the x-axis nd z-axis
% time - simulation time signal
% z_warm - initial guess of the decision variables which are stacked vertically as
%          a collected variables vector, consist of the state and control
%          variables and the slack variables z_warm = [u_warm^T, x_warm^T,
%          s_warm^T]^T
%
% OUTPUT
% force_top  - required cable tension of the top cable, along with the
%              negative x-axis direction
% force_btm  - required cable tension of the bottom cable, along with the
%              positive x-axis direction
% force_right - required cable tension of the riht cable, along with the
%              positive z-axis direction
% force_left - required cable tension of the left cable, along with the
%              negative z-axis direction
% z_last   - the decision variables at last instance, used for warmstarting
%            the SQP.
% flag   - an integer that describes the exit condition of SQP. 1
%          represents function converged to the solution x within maximum iteration,
%          and 0 represents the SQP algorithm can not find a solution within maximum
%          iteration.
%
%
% Developed by Yongjun Yan. Updated Feb 2024.
global pos
%% Initialization SQP
Horizon = 0.1;
Samp_time = 0.01; 
Samp_Crt = 0.05;
Num = Horizon/Samp_time;
DurCrt = Samp_Crt/Samp_time;
NumCrt = Num/DurCrt;
size_x = 3;                   % number of states
size_u = 4;                   % number of control input
size_C = 9;
size_Cbar = 6;
opt.itmax = 10; % maximum iteration of the SQP
opt.tol = 10e-4; % convergence tolerance of SQP
opt.gamma = 10;   % weight of slack variable 
opt.intTol = 1e-4;
opt.display = 'off';
opt.iterplot = false;
opt.gap = false;
% uu = [0.001, 0.001, 0.5008, 0.001]; % umcomment to generate the initial state
% uu = repmat(uu,1,Num);
% xx = [-0.1363,-0.3840,-0.0157];
% xx = repmat(xx,1,Num);
% s = zeros(Num,1);
% z = [reshape(uu,[size_u*Num,1]);reshape(xx,[size_x*Num,1]);s];
% z_last = zeros(80,1);
lambda = zeros(size_x*Num,1);   % initial guess of dual variables
nu = zeros(Num*(size_C+size_Cbar+1),1);   % initial guess of dual variables
km.z = z_warm;
km.l = lambda;
km.v = nu;
trq_right_1_ori = 0;
trq_btm_2_ori = 0;
trq_top_3_ori = 0;
trq_left_4_ori = 0;
% tip_pos_orie_last = xsim(:,1);

%% Reconstruction of the (x_0, u_0) vector
SSMDim = 3;
overEmbed = 0;
% [yData, opts_embd] = coordinatesEmbeddingControl(dataAss, SSMDim, 'OverEmbedding', overEmbed);
x_0 = obs2lowdim_func(dataAss(1),dataAss(2),dataAss(3));
% x_0 = Vde*yData;
% x_0 = [0.0566014740565661; -0.200148373213334; -0.0240715398307494];
% uu = reshape(km.z(1:size_u*Num,1),[size_u,Num]);
% u_0 = [uu(1,1);bending_direction];
if time < 5.5
    trq_right_1 = 0;
    trq_btm_2 = 0;
    trq_top_3 = 0;
    trq_left_4 = 0;
    flag = 0;
    z_last = z_warm;
elseif time < 12.45
    trq_right_1 = 963/1000;
    trq_btm_2 = 457/1000;
    trq_top_3 = 1580/1000;
    trq_left_4 = 984/1000;
    flag = 0;
    z_last = z_warm;
elseif time > 39
    trq_right_1 = 0;
    trq_btm_2 = 0;
    trq_top_3 = 0;
    trq_left_4 = 0;
    flag = 0;
    z_last = z_warm;
else
    %% Get the position and velocity information (sequence) over the horizon
    step = fix((time-5.5)/Samp_time);
    % step = fix(rem(step,350));
    ref_pos = pos(step+1:step+(Num-1)+1,1:3)'; % Give the position of the current predictive horizon, unit: mm
    ref_crt = pos(step+1,4:7)'; % Give the velocity of the current predictive horizon, unit: mm
    
    p = ref_pos; % Parameter comprise slope data and reference speed vector
    %% Solve the optimal control problem
    der = struct('Cu',zeros(size_C,size_u,Num),'Cbarx',zeros(size_Cbar,size_x,Num),'fu',zeros(size_x,size_u,Num),'fx',zeros(size_x,size_x,Num-1),'Lx',zeros(1,size_x,Num),'Phix',zeros(1,size_x,Num),'Lu',zeros(1,size_u,Num),'Luu',zeros(size_u,size_u,Num),'Lxu',zeros(size_u,size_x,Num),'Lxx',zeros(size_x,size_x,Num-1),'Phixx',zeros(size_x,size_x,Num));
    % tic
    [x, val, flag] = SeqQuadProg(x_0, km,opt,size_x,size_u,p,Num,der);
    % [x, val, flag] = seq_quad_prog(x_0, km,opt,size_x,size_u,size_C,size_Cbar,p,Num,der);
    % time(i) = toc;
    z_last = x;
    % z_last = z_warm;
    uu = reshape(x(1:size_u*Num,1),[size_u,Num]);
    trq_right_1_ori = uu(1,10);
    trq_btm_2_ori = uu(2,10);
    trq_top_3_ori = uu(3,10);
    trq_left_4_ori = uu(4,10);
    % trq_right_1 = trq_right_1_ori;
    % trq_btm_2 = trq_btm_2_ori;
    % trq_top_3 = trq_top_3_ori;
    % trq_left_4 = trq_left_4_ori;
    threshold = 0.2;
    if (trq_right_1_ori < ref_crt(1) + threshold) && (trq_right_1_ori > ref_crt(1) - threshold)
        trq_right_1 = trq_right_1_ori;
    else
        trq_right_1 = ref_crt(1);
    end
    if (trq_btm_2_ori < ref_crt(2) + threshold) && (trq_btm_2_ori > ref_crt(2) - threshold)
        trq_btm_2 = trq_btm_2_ori;
    else
        trq_btm_2 = ref_crt(2);
    end
    if (trq_top_3_ori < ref_crt(3) + threshold) && (trq_top_3_ori > ref_crt(3) - threshold)
        trq_top_3 = trq_top_3_ori;
    else
        trq_top_3 = ref_crt(3);
    end
    if (trq_left_4_ori < ref_crt(4) + threshold) && (trq_left_4_ori > ref_crt(4) - threshold)
        trq_left_4 = trq_left_4_ori;
    else
        trq_left_4 = ref_crt(4);
    end
    % if trq_right_1_Ori > trq_left_4_Ori
    %     trq_right_1 = trq_right_1_Ori - trq_left_4_Ori;
    %     trq_left_4 = 0;
    % else
    %     trq_left_4 = trq_left_4_Ori - trq_right_1_Ori;
    %     trq_right_1 = 0;
    % end
    % if abs(trq_right_1 - trq_right_1_last) > 0.3
    %     trq_right_1 = trq_right_1_last;
    % end
    % if abs(trq_btm_2 - trq_btm_2_last) > 0.3
    %     trq_btm_2 = trq_btm_2_last;
    % end
    % if abs(trq_top_3 - trq_top_3_last) > 0.3
    %     trq_top_3 = trq_top_3_last;
    % end
    % if abs(trq_left_4 - trq_left_4_last) > 0.3
    %     trq_left_4 = trq_left_4_last;
    % end
end
end
